simulink model "GDFLIB_FilterFIR_BAM_F32"  (Simulink 7.3)
settings: Solver=ode45  StartTime=0.0  StopTime=10.0  RelTol=1e-3
undefined symbols (not defined in the file): pf32CoefBuf, u32Order
settings Model: Creator=RE004C  LastModifiedBy=RE004C
settings HardwareCC: ProdIntDivRoundTo=Zero  ProdEndianess=BigEndian  ProdHWDeviceType=Freescale->32-bit PowerPC

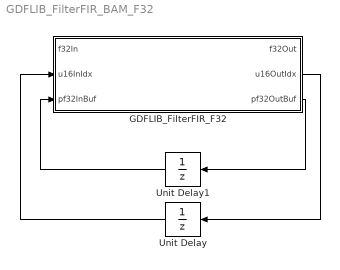
== system GDFLIB_FilterFIR_BAM_F32 ==
  GDFLIB_FilterFIR_F32 : Subsystem  mask(GDFLIB_FilterFIR_F32){u32Order=u32Order, pf32CoefBuf=pf32CoefBuf}
      mask help: Bit accurate model of FIR filter. All parameters as well as input and output are 32bit integers.
      mask init:
      | pos = get_param(gcb, 'Position');width = pos(3) - pos(1); height = pos(4) - pos(2);tX=width/2;tY=height*0.9;
      mask Display:
      | color('black');
      | port_label('input',1,'f32In');
      | port_label('input',2,'u16InIdx');
      | port_label('input',3,'pf32InBuf');
      | port_label('output',1,'f32Out');
      | port_label('output',2,'u16OutIdx');
      | port_label('output',3,'pf32OutBuf');
      | color('black');
      | disp('GDFLIB_FilterFIR_F32');
      | color('blue');
      | text(tX,tY, 'BAM', 'horizontalAlignment', 'center');
  Unit Delay : UnitDelay  SampleTime=-1
  Unit Delay1 : UnitDelay  SampleTime=-1
  wires:
  GDFLIB_FilterFIR_F32/2(u16OutIdx) -> Unit Delay/1
  Unit Delay/1 -> GDFLIB_FilterFIR_F32/2(u16InIdx)
  GDFLIB_FilterFIR_F32/3(pf32OutBuf) -> Unit Delay1/1
  Unit Delay1/1 -> GDFLIB_FilterFIR_F32/3(pf32InBuf)

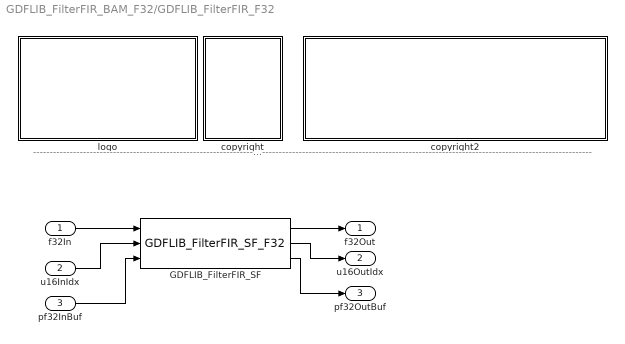
== system GDFLIB_FilterFIR_BAM_F32/GDFLIB_FilterFIR_F32 ==
  note: ---------------------------------------------------------------------------------------------------------------------------------------------------------------------------------------------------
  f32In : Inport  OutDataType=fixdt(1, 16)  OutScaling=2^0
  u16InIdx : Inport  Port=2  OutDataType=fixdt(1, 16)  OutScaling=2^0
  pf32InBuf : Inport  Port=3  OutDataType=fixdt(1, 16)  OutScaling=2^0
  GDFLIB_FilterFIR_SF : S-Function  FunctionName=GDFLIB_FilterFIR_SF_F32  Parameters=u32Order,pf32CoefBuf  EnableBusSupport=off
  copyright : Subsystem
      mask Display: text(10,90,'FILE:');text(10,75,'DESRIPTION:')text(10,60,'COPYRIGHT:')text(10,45,'VERSION:')text(10,30,'DATE:')
  copyright2 : Subsystem
      mask Display: text(10,90,'GDFLIB_FilterFIR_BAM_F32.mdl');text(10,75,'FIR filter.');text(10,60,'Freescale')text(10,45,'0.1');text(10,30,'20-Sep-2011');
  logo : Subsystem
      mask Display: image(imread('logo.jpg'))
  f32Out : Outport  OutDataType=fixdt(1, 16)  OutScaling=2^0
  u16OutIdx : Outport  Port=2  OutDataType=fixdt(1, 16)  OutScaling=2^0
  pf32OutBuf : Outport  Port=3  OutDataType=fixdt(1, 16)  OutScaling=2^0
  wires:
  f32In/1 -> GDFLIB_FilterFIR_SF/1
  GDFLIB_FilterFIR_SF/1 -> f32Out/1
  u16InIdx/1 -> GDFLIB_FilterFIR_SF/2
  pf32InBuf/1 -> GDFLIB_FilterFIR_SF/3
  GDFLIB_FilterFIR_SF/2 -> u16OutIdx/1
  GDFLIB_FilterFIR_SF/3 -> pf32OutBuf/1

== system GDFLIB_FilterFIR_BAM_F32/GDFLIB_FilterFIR_F32/copyright ==

== system GDFLIB_FilterFIR_BAM_F32/GDFLIB_FilterFIR_F32/copyright2 ==

== system GDFLIB_FilterFIR_BAM_F32/GDFLIB_FilterFIR_F32/logo ==
